simulink model "adbad_main"  (R2017b)
settings: Solver=VariableStepAuto  StartTime=0.0  StopTime=1000  RelTol=1e-3
undefined symbols (not defined in the file): sigbuilder_block
settings Model: Creator=uidn7735  LastModifiedBy=uidn7735

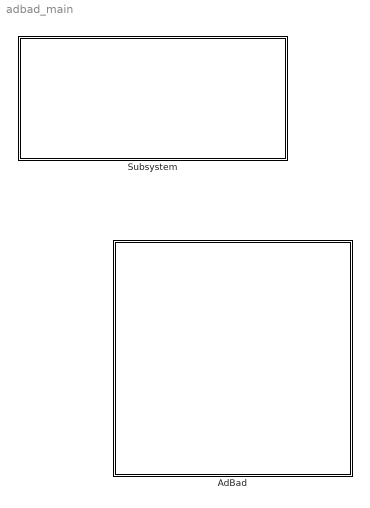
== system adbad_main ==
  AdBad : Subsystem
  Subsystem : Subsystem

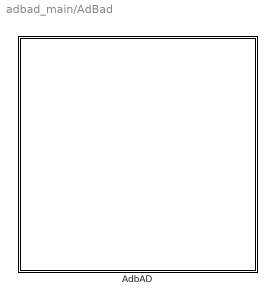
== system adbad_main/AdBad ==
  AdbAD : Stateflow chart  TreatAsAtomicUnit=on

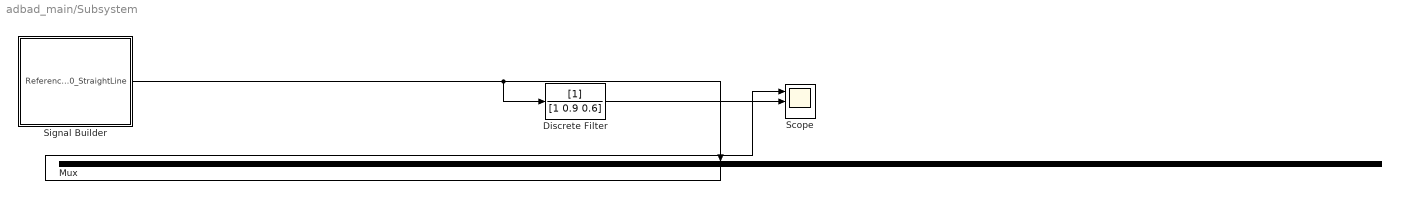
== system adbad_main/Subsystem ==
  Discrete Filter : DiscreteFilter  Denominator=[1 0.9 0.6]  SampleTime=0.01
  Mux : Mux  Inputs=1
  Scope : Scope  NumInputPorts=3
  Signal Builder : Subsystem  Tag=STV Subsys  LoadFcn=sigbuilder_block('load');  StartFcn=sigbuilder_block('start');  StopFcn=sigbuilder_block('stop');  ClipboardFcn=sigbuilder_block('clipboard');  mask(Sigbuilder block){tuvar=[0:10]}
      mask help: Simulink:masks:SigbuilderBlock_MD
      mask init:
      | if ~strcmp(get_param(bdroot(gcbh),'SimulationStatus'),'stopped') tuvar = sigbuilder_block('maskInit'); end
      settings: CopyFcn=sigbuilder_block('copy');  DeleteFcn=sigbuilder_block('delete');  ModelCloseFcn=sigbuilder_block('modelClose');  PreSaveFcn=sigbuilder_block('preSave');  PauseFcn=sigbuilder_block('pause');  ContinueFcn=sigbuilder_block('continue');  NameChangeFcn=sigbuilder_block('namechange');  OpenFcn=sigbuilder_block('open',[6 30 1428 682.5 ]);  CloseFcn=sigbuilder_block('close');
      mask Display: plot(0, 0, 100, 100,[2, 2, 32, 32, 2], [68, 8, 8, 68, 68],[32, 2], [38, 38], [32, 19, 2],[53, 60, 44], [32, 17, 17, 2],[16, 16, 31, 31]);txt = getActiveGroup(gcbh);text(2, 100, txt,'verticalAlignment', 'top');
  wires:
  Mux/1 -> Scope/1
  Signal Builder/1(ReferenceRoad_00_StraightLine) -> Discrete Filter/1, Mux/1
  Discrete Filter/1 -> Scope/2

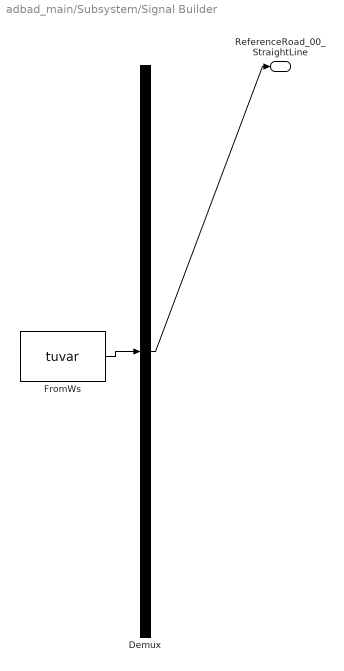
== system adbad_main/Subsystem/Signal Builder ==
  Demux : Demux  Tag=STV Demux  Outputs=1
  FromWs : FromWorkspace  Tag=STV FromWs  VariableName=tuvar  SampleTime=0
      SigBuilderData=|
      | common.afterFinalStr = 'Extrapolate'
      | common.sampleTime = 0
      | dataSet.timeRange = [0 1000]
      | dataSet.name = 'Group 1'
      | sbobj.Groups.Name = 'Group 1'
      | sbobj.Groups.Signals.Name = 'ReferenceRoad_00_StraightLine'
      | sbobj.Groups.Signals.XData = [0 6 26 40 58 86 112 120 134 148 168 168 206 206 236 270 306 330 368 406 446 470 486 506 522 542 570 584 606 618 638 658 682 696 706 738 776 806 822 834 850 870 906 924 938 958 976 1000]
      | sbobj.Groups.Signals.YData = [0.53 0.53 0.725 1.575 1.605 1.85 1.605 1.86 1.685 1.725 1.25 1.245 1.245 1.25 1.205 0.995 0.98 1.155 0.36 0.31 0.515 0.075 0.19 -0.06 -0.065 -0.205 -0.095 0.19 -0.115 -0.06 0.22 0.125 0.475 0.295 0.335 0.55 0.325 0.665 0.67 1.06 1.07 0.67 0.67 0.515 0.625 0.155 0.11 -0.0838461538462]
      | sbobj.Groups.TimeRange = [0 1000]
  ReferenceRoad_00_StraightLine : Outport  Tag=STV Outport
  wires:
  FromWs/1 -> Demux/1
  Demux/1 -> ReferenceRoad_00_StraightLine/1

== stateflow chart adbad_main/AdBad/AdbAD ==
